simulink model "RBDmodel"  (R2023a)
settings: Solver=ode15s  StartTime=0.0  StopTime=4  FixedStep=0.0001  RelTol=1e-3  AbsTol=1e-3  EnableMultiTasking=on
model workspace (MAT data in the model file):
  C_Gimbal = 0.5
  C_IAP = 0.01
  IAP_Pa = 0
  K_Gimbal = 0
  K_IAP = 200
  LeftAbdominalMuscleForce = 0
  LeftBackMuscleForce = 0
  LeftTransverse1MuscleForce = 0
  LeftTransverse2MuscleForce = 0
  Moment_AR = 0
  Moment_FE = 7.5
  Moment_LB = 0
  RightAbdominalMuscleForce = 0
  RightBackMuscleForce = 0
  RightTransverse1MuscleForce = 0
  RightTransverse2MuscleForce = 0
  a = 1
  b = 1
  muscle_color = [0 0 1]
  muscle_radius = 1
undefined symbols (not defined in the file): X, Y, Z
libraries: nesl_utility x346, sm_lib x329, simulink_extras x33, checkpacklib x3, simulink x1
(part 1 of 12)
settings Model: PacingRate=0.110000  Creator=Siril TD  LastModifiedBy=siril
settings SolverCC: ZeroCrossAlgorithm=Adaptive  AutoInsertRateTranBlk=on
settings DataIOCC: LimitDataPoints=on  MaxDataPoints=50000  ReturnWorkspaceOutputsName=SDOSimTest_Log
settings OptimizationCC: LifeSpan=inf
settings DebuggingCC: IgnoredZcDiagnostic=none  UnconnectedInputMsg=warning  UnconnectedOutputMsg=warning  UnconnectedLineMsg=warning  AllowSymbolicDim=off  SFUnexpectedBacktrackingDiag=warning  SFNoUnconditionalDefaultTransitionDiag=warning  SFExecutionAtInitializationDiag=none  ArithmeticOperatorsInVariantConditions=warning
settings ModelReferenceCC: EnableRefExpFcnMdlSchedulingChecks=on
settings SFSimCC: SimUseLocalCustomCode=off  CustomCodeUndefinedFunction=UseInterfaceOnly
settings RTWCC: RTWUseLocalCustomCode=off  DLArmComputeVersion=19.05
settings CodeAppCC: StateflowObjectComments=on
settings GRTTargetCC: TargetLangStandard=C89/C90 (ANSI)
settings ConfigComp: CovMetricSettings=dw  CovSaveCumulativeToWorkspaceVar=on  CovSaveSingleToWorkspaceVar=on  CovExternalEMLEnable=off  CovSFcnEnable=off
settings SimscapeCC: SimscapeLogType=all  SimscapeLogSimulationStatistics=on  SimscapeLogDataHistory=10000

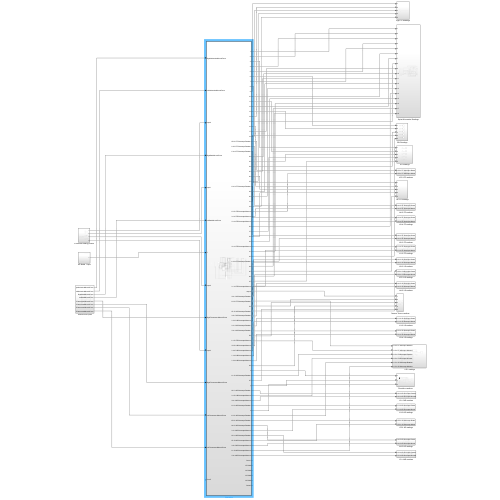
[thumbnail: Simulink's stored preview of the top-level diagram]
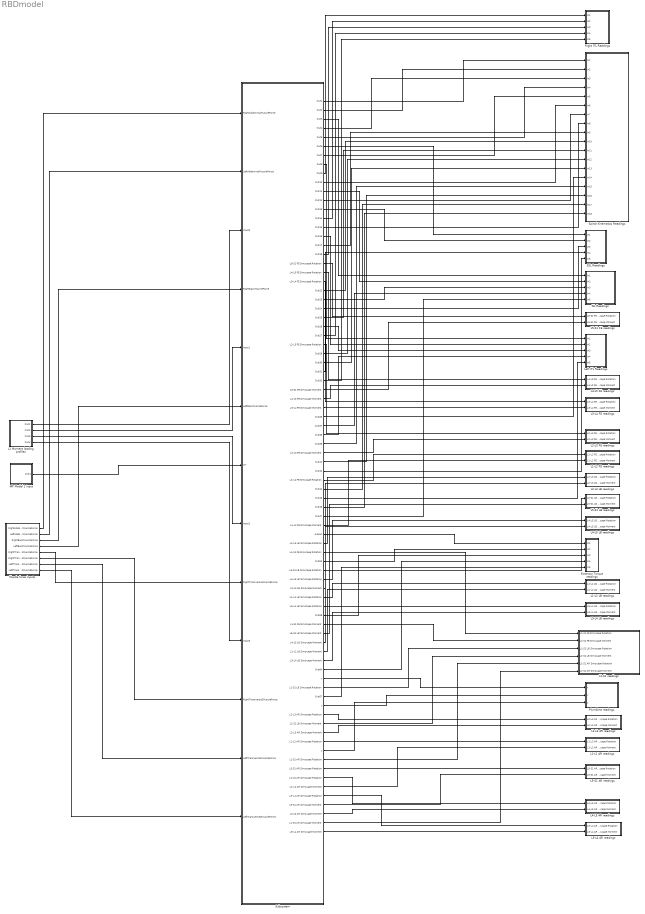
== system RBDmodel ==
  Extensor Torque readings : Subsystem
  IAP Model 1 input : Subsystem
  ISL Readings : Subsystem
  L1 Moment loading profiles : Subsystem
  L1-L2 AR readings : Subsystem
  L1-L2 FE readings : Subsystem
  L1-L2 LB readings : Subsystem
  L1-S1 readings : Subsystem
  L2-L3 AR readings : Subsystem
  L2-L3 FE readings : Subsystem
  L2-L3 LB readings : Subsystem
  L3-L4 AR readings : Subsystem
  L3-L4 FE readings : Subsystem
  L3-L4 LB readings : Subsystem
  L4-L5 AR readings : Subsystem
  L4-L5 FE readings : Subsystem
  L4-L5 LB readings : Subsystem
  L5-S1 AR readings : Subsystem
  L5-S1 FE readings : Subsystem
  L5-S1 LB readings : Subsystem
  Left ITL Readings : Subsystem
  Muscle force inputs : Subsystem
  Plumbline readings : Subsystem
  Right ITL Readings : Subsystem
  SSL Readings : Subsystem
  Spinal Kinematics Readings : Subsystem
  Subsystem : Subsystem  TreatAsAtomicUnit=on
  wires:
  Subsystem/20(L4-L5 FE Simscape Rotation) -> L4-L5 FE readings/1(L4-L5 FE Simscape Rotation)
  Subsystem/67(Out67) -> Extensor Torque readings/5(In5)
  Muscle force inputs/4(LeftBackMuscleForce) -> Subsystem/6(LeftBackMuscleForce)
  Muscle force inputs/3(RightBackMuscleForce) -> Subsystem/4(RightBackMuscleForce)
  L1 Moment loading profiles/1(Out1) -> Subsystem/3(input0)
  Subsystem/31(Out31) -> SSL Readings/4(In4)
  Subsystem/81(L1-S1 AR Simscape Moment) -> L1-S1 readings/6(L1-S1 AR Simscape Moment)
  Subsystem/56(L1-L2 LB Simscape Rotation) -> L1-L2 LB readings/1(L1-L2 LB Simscape Rotation)
  L1 Moment loading profiles/2(Out2) -> Subsystem/5(input1)
  L1 Moment loading profiles/3(Out3) -> Subsystem/8(input2)
  Subsystem/50(L2-L3 LB Simscape Rotation) -> L2-L3 LB readings/1(L2-L3 LB Simscape Rotation)
  Subsystem/6(Out6) -> SSL Readings/1(In1)
  L1 Moment loading profiles/4(Out4) -> Subsystem/10(input3)
  Muscle force inputs/1(RightAbdominalMuscleForce) -> Subsystem/1(RightAbdominalMuscleForce)
  Subsystem/16(Out16) -> Left ITL Readings/2(In2)
  IAP Model 1 input/1(Out1) -> Subsystem/7(In7)
  Muscle force inputs/2(LeftAbdominalMuscleForce) -> Subsystem/2(LeftAbdominalMuscleForce)
  Muscle force inputs/5(RightTransverse1MuscleForce) -> Subsystem/9(RightTransverse1MuscleForce)
  Muscle force inputs/6(RightTransverse2MuscleForce) -> Subsystem/11(RightTransverse2MuscleForce)
  Subsystem/62(L1-L2 LB Simscape Moment) -> L1-L2 LB readings/2(L1-L2 LB Simscape Moment)
  Muscle force inputs/8(LeftTransverse2MuscleForce) -> Subsystem/13(LeftTransverse2MuscleForce)
  Muscle force inputs/7(LeftTransverse1MuscleForce) -> Subsystem/12(LeftTransverse1MuscleForce)
  Subsystem/63(L3-L4 LB Simscape Moment) -> L3-L4 LB readings/2(L3-L4 LB Simscape Moment)
  Subsystem/1(Out1) -> Spinal Kinematics Readings/1(In1)
  Subsystem/30(Out30) -> Spinal Kinematics Readings/13(In13)
  Subsystem/2(Out2) -> Spinal Kinematics Readings/2(In2)
  Subsystem/13(Out13) -> SSL Readings/2(In2)
  Subsystem/21(L3-L4 FE Simscape Rotation) -> L3-L4 FE readings/1(L3-L4 FE Simscape Rotation)
  Subsystem/3(Out3) -> ISL Readings/1(In1)
  Subsystem/44(Out44) -> Spinal Kinematics Readings/17(In17)
  Subsystem/25(Out25) -> Spinal Kinematics Readings/11(In11)
  Subsystem/79(L5-S1 AR Simscape Moment) -> L5-S1 AR readings/2(L5-S1 AR Simscape Moment)
  Subsystem/4(Out4) -> Spinal Kinematics Readings/3(In3)
  Subsystem/5(Out5) -> Spinal Kinematics Readings/4(In4)
  Subsystem/77(L1-L2 AR Simscape Moment) -> L1-L2 AR readings/2(L1-L2 AR Simscape Moment)
  Subsystem/36(Out36) -> Spinal Kinematics Readings/14(In14)
  Subsystem/78(L3-L4 AR Simscape Rotation) -> L3-L4 AR readings/1(L3-L4 AR Simscape Rotation)
  Subsystem/26(Out26) -> Left ITL Readings/3(In3)
  Subsystem/7(Out7) -> Spinal Kinematics Readings/5(In5)
  Subsystem/18(Out18) -> Right ITL Readings/3(In3)
  Subsystem/8(Out8) -> Left ITL Readings/1(In1)
  Subsystem/9(Out9) -> Right ITL Readings/1(In1)
  Subsystem/10(Out10) -> Spinal Kinematics Readings/6(In6)
  Subsystem/11(Out11) -> ISL Readings/2(In2)
  Subsystem/12(Out12) -> Spinal Kinematics Readings/7(In7)
  Subsystem/38(Out38) -> Left ITL Readings/4(In4)
  Subsystem/14(Out14) -> Right ITL Readings/2(In2)
  Subsystem/15(Out15) -> Spinal Kinematics Readings/8(In8)
  Subsystem/17(Out17) -> Spinal Kinematics Readings/9(In9)
  Subsystem/27(Out27) -> Right ITL Readings/4(In4)
  Subsystem/19(L5-S1 FE Simscape Rotation) -> L5-S1 FE readings/1(L5-S1 FE Simscape Rotation)
  Subsystem/22(Out22) -> Spinal Kinematics Readings/10(In10)
  Subsystem/33(L5-S1 FE Simscape Moment) -> L5-S1 FE readings/2(L5-S1 FE Simscape Moment)
  Subsystem/23(Out23) -> ISL Readings/3(In3)
  Subsystem/45(Out45) -> Left ITL Readings/5(In5)
  Subsystem/24(Out24) -> SSL Readings/3(In3)
  Subsystem/28(L2-L3 FE Simscape Rotation) -> L2-L3 FE readings/1(L2-L3 FE Simscape Rotation)
  Subsystem/29(Out29) -> Spinal Kinematics Readings/12(In12)
  Subsystem/32(Out32) -> Right ITL Readings/5(In5)
  Subsystem/34(L4-L5 FE Simscape Moment) -> L4-L5 FE readings/2(L4-L5 FE Simscape Moment)
  Subsystem/59(L1-S1 FE Simscape Moment) -> L1-S1 readings/2(L1-S1 FE Simscape Moment)
  Subsystem/35(L3-L4 FE Simscape Moment) -> L3-L4 FE readings/2(L3-L4 FE Simscape Moment)
  Subsystem/37(Out37) -> ISL Readings/4(In4)
  Subsystem/51(L1-S1 FE Simscape Rotation) -> L1-S1 readings/1(L1-S1 FE Simscape Rotation)
  Subsystem/39(Out39) -> Spinal Kinematics Readings/15(In15)
  Subsystem/40(L2-L3 FE Simscape Moment) -> L2-L3 FE readings/2(L2-L3 FE Simscape Moment)
  Subsystem/41(Out41) -> Spinal Kinematics Readings/16(In16)
  Subsystem/42(Out42) -> SSL Readings/5(In5)
  Subsystem/43(L1-L2 FE Simscape Rotation) -> L1-L2 FE readings/1(L1-L2 FE Simscape Rotation)
  Subsystem/46(Out46) -> Spinal Kinematics Readings/18(In18)
  Subsystem/47(Out47) -> ISL Readings/5(In5)
  Subsystem/48(L1-L2 FE Simscape Moment) -> L1-L2 FE readings/2(L1-L2 FE Simscape Moment)
  Subsystem/49(output) -> Extensor Torque readings/1(In1)
  Subsystem/52(Out52) -> Extensor Torque readings/2(In2)
  Subsystem/68(y) -> Plumbline readings/2(y)
  Subsystem/53(L5-S1 LB Simscape Rotation) -> L5-S1 LB readings/1(L5-S1 LB Simscape Rotation)
  Subsystem/54(L4-L5 LB Simscape Rotation) -> L4-L5 LB readings/1(L4-L5 LB Simscape Rotation)
  Subsystem/55(L2-L3 LB Simscape Moment) -> L2-L3 LB readings/2(L2-L3 LB Simscape Moment)
  Subsystem/57(L3-L4 LB Simscape Rotation) -> L3-L4 LB readings/1(L3-L4 LB Simscape Rotation)
  Subsystem/58(Out58) -> Extensor Torque readings/3(In3)
  Subsystem/60(L5-S1 LB Simscape Moment) -> L5-S1 LB readings/2(L5-S1 LB Simscape Moment)
  Subsystem/61(L4-L5 LB Simscape Moment) -> L4-L5 LB readings/2(L4-L5 LB Simscape Moment)
  Subsystem/64(Out64) -> Extensor Torque readings/4(In4)
  Subsystem/65(x) -> Plumbline readings/1(x)
  Subsystem/66(L1-S1 LB Simscape Rotation) -> L1-S1 readings/3(L1-S1 LB Simscape Rotation)
  Subsystem/69(L2-L3 AR Simscape Rotation) -> L2-L3 AR readings/1(L2-L3 AR Simscape Rotation)
  Subsystem/70(L1-S1 LB Simscape Moment) -> L1-S1 readings/4(L1-S1 LB Simscape Moment)
  Subsystem/71(L2-L3 AR Simscape Moment) -> L2-L3 AR readings/2(L2-L3 AR Simscape Moment)
  Subsystem/72(L1-L2 AR Simscape Rotation) -> L1-L2 AR readings/1(L1-L2 AR Simscape Rotation)
  Subsystem/73(z) -> Plumbline readings/3(z)
  Subsystem/74(L1-S1 AR Simscape Rotation) -> L1-S1 readings/5(L1-S1 AR Simscape Rotation)
  Subsystem/75(L5-S1 AR Simscape Rotation) -> L5-S1 AR readings/1(L5-S1 AR Simscape Rotation)
  Subsystem/76(L4-L5 AR Simscape Rotation) -> L4-L5 AR readings/1(L4-L5 AR Simscape Rotation)
  Subsystem/80(L4-L5 AR Simscape Moment) -> L4-L5 AR readings/2(L4-L5 AR Simscape Moment)
  Subsystem/82(L3-L4 AR Simscape Moment) -> L3-L4 AR readings/2(L3-L4 AR Simscape Moment)

== system RBDmodel/Extensor Torque readings ==
  In1 : Inport
  In2 : Inport  Port=2
  In3 : Inport  Port=3
  In4 : Inport  Port=4
  In5 : Inport  Port=5
  Display{,1..4} (5 alike) : Display
      settings: Decimation=2
  Gain{9,11..14} (5 alike) : Gain
  IAP Extensor Torque at L1-L2 : Scope
  IAP Extensor Torque at L2-L3 (reported) : Scope
  IAP Extensor Torque at L3-L4 : Scope
  IAP Extensor Torque at L4-L5 : Scope
  IAP Extensor Torque at L5-S1 : Scope
  wires:
  Gain11/1 -> Display1/1
  Gain9/1 -> Display/1
  In5/1 -> Gain14/1, IAP Extensor Torque at L5-S1/1
  In2/1 -> Gain9/1, IAP Extensor Torque at L2-L3 (reported)/1
  Gain12/1 -> Display2/1
  In4/1 -> Gain13/1, IAP Extensor Torque at L4-L5/1
  In3/1 -> Gain12/1, IAP Extensor Torque at L3-L4/1
  Gain13/1 -> Display3/1
  In1/1 -> Gain11/1, IAP Extensor Torque at L1-L2/1
  Gain14/1 -> Display4/1

== system RBDmodel/IAP Model 1 input ==
  Constant96 : Constant  Value=IAP_Pa
  Out1 : Outport
  wires:
  Constant96/1 -> Out1/1

== system RBDmodel/ISL Readings ==
  In1 : Inport
  In2 : Inport  Port=2
  In3 : Inport  Port=3
  In4 : Inport  Port=4
  In5 : Inport  Port=5
  L1-L2 ISL force : Scope
  L2-L3 ISL force : Scope
  L3-L4 ISL force : Scope
  L4-L5 ISL force : Scope
  L5-S1 ISL force : Scope
  wires:
  In4/1 -> L5-S1 ISL force/1
  In2/1 -> L2-L3 ISL force/1
  In1/1 -> L1-L2 ISL force/1
  In3/1 -> L3-L4 ISL force/1
  In5/1 -> L4-L5 ISL force/1

== system RBDmodel/L1 Moment loading profiles ==
  Gain10 : Gain  Gain=-1
  Horizontal force at T1 : simulink/Sources/Ramp  slope=0  start=0  InitialOutput=0
  Moment_AR : Sin  Amplitude=Moment_AR  SampleTime=0
  Moment_FE : Sin  Amplitude=-Moment_FE  SampleTime=0
  Moment_LB : Sin  Amplitude=-Moment_LB  SampleTime=0
  Scope2 : Scope
  Out1 : Outport
  Out2 : Outport  Port=2
  Out3 : Outport  Port=3
  Out4 : Outport  Port=4
  wires:
  Gain10/1 -> Scope2/1
  Horizontal force at T1/1 -> Out4/1
  Moment_LB/1 -> Out2/1
  Moment_AR/1 -> Out1/1
  Moment_FE/1 -> Gain10/1, Out3/1

== system RBDmodel/L1-L2 AR readings ==
  L1-L2 AR Simscape Rotation : Inport
  L1-L2 AR Simscape Moment : Inport  Port=2
  L1-L2 AR Moment : Scope
  L1-L2 AR Rotation : Scope
  L1-L2 AR Simscape : Record  FileSettingsInternal="{\"entries\":[{\"content\":{\"excelSettings\":{\"content\":{},\"type\":\"Streamout.ExcelSettings\"}},\"type\":\"Streamout.FileSettingStorage\",\"uuid\":\"b28dc066-991e-4613-a00d-d29ff6d798a1\"}],\"packageUris\":[\"http://schema.mathworks.com/mf0/streamout_blocks/R2020a\"],\"version\":\"1.0\"}"  Layout=[1 1]  SignalsInternal="{\"entries\":[{\"content\":{\"signals\":[{\"content\":{\"blockPath\":[\"RBDmodel/L1-L2 AR readings/L1-L2 AR Simscape\"],\"dimensions\":[1],\"domain\":\"RBDmodel/L1-L2 AR readings/L1-L2 AR Simscape\",\"lineColor\":\"#ff6929\",\"port\":1,\"sid\":[\"\"],\"signalID\":1360,\"signalName\":\"L1-L2 AR Simscape Rotation\"},\"type\":\"RecordBlkView.Signal\",\"uuid\":\"8ba76c58-794a-4c9e-a7b1-df05cf77fcb8\"},{\"content\":{\"blockPath\":[\"RBDmodel/L1-L2 AR readings/L1-L2 AR Simscape\"],\"dimensions\":[1],\"domain\":\"RBDmodel/L1-L2 AR readings/L1-L2 AR Simscape\",\"lineColor\":\"#b746ff\",\"port\":2,\"sid\":[\"\"],\"signalID\":1364,\"signalName\":\"L1-L2 AR Simscape Moment\"},\"type\":\"RecordBlkView.Signal\",\"uuid\":\"7d4a0f01-01c2-4817-9b83-8632446fab25\"}]},\"type\":\"RecordBlkView.InputSignals\",\"uuid\":\"3a315800-566e-4bdd-9ec3-69dc347d5a26\"}],\"packageUris\":[\"http://schema.mathworks.com/mf0/streamout_blocks/R2020a\"],\"version\":\"1.0\"}"  VisualizationBindings="{\"xyplotplugin\":{\"info\":[{\"series\":[],\"subplotID\":1}]}}"  CompatibilityTag=XY
  wires:
  L1-L2 AR Simscape Rotation/1 -> L1-L2 AR Simscape/1, L1-L2 AR Rotation/1
  L1-L2 AR Simscape Moment/1 -> L1-L2 AR Simscape/2, L1-L2 AR Moment/1

== system RBDmodel/L1-L2 FE readings ==
  L1-L2 FE Simscape Rotation : Inport
  L1-L2 FE Simscape Moment : Inport  Port=2
  L1-L2 FE Moment : Scope
  L1-L2 FE Rotation : Scope
  L1-L2 FE Simscape : Record  FileSettingsInternal="{\"entries\":[{\"content\":{\"excelSettings\":{\"content\":{},\"type\":\"Streamout.ExcelSettings\"}},\"type\":\"Streamout.FileSettingStorage\",\"uuid\":\"8ce7ea1e-727d-4085-a2f9-c3a4a6f5bb0a\"}],\"packageUris\":[\"http://schema.mathworks.com/mf0/streamout_blocks/R2020a\"],\"version\":\"1.0\"}"  Layout=[1 1]  SignalsInternal="{\"entries\":[{\"content\":{\"signals\":[{\"content\":{\"blockPath\":[\"RBDmodel/L1-L2 FE readings/L1-L2 FE Simscape\"],\"dimensions\":[1],\"domain\":\"RBDmodel/L1-L2 FE readings/L1-L2 FE Simscape\",\"lineColor\":\"#64d413\",\"port\":1,\"sid\":[\"\"],\"signalID\":1368,\"signalName\":\"L1-L2 FE Simscape Rotation\"},\"type\":\"RecordBlkView.Signal\",\"uuid\":\"2003be24-72ea-4258-88d8-cae005e22d9e\"},{\"content\":{\"blockPath\":[\"RBDmodel/L1-L2 FE readings/L1-L2 FE Simscape\"],\"dimensions\":[1],\"domain\":\"RBDmodel/L1-L2 FE readings/L1-L2 FE Simscape\",\"lineColor\":\"#ff13a6\",\"port\":2,\"sid\":[\"\"],\"signalID\":1372,\"signalName\":\"L1-L2 FE Simscape Moment\"},\"type\":\"RecordBlkView.Signal\",\"uuid\":\"2512a7a8-a368-412a-aefb-8db868f0d60c\"}]},\"type\":\"RecordBlkView.InputSignals\",\"uuid\":\"ac10ff46-4b91-49cb-b675-363e0bf05791\"}],\"packageUris\":[\"http://schema.mathworks.com/mf0/streamout_blocks/R2020a\"],\"version\":\"1.0\"}"  VisualizationBindings="{\"xyplotplugin\":{\"info\":[{\"series\":[],\"subplotID\":1}]}}"  CompatibilityTag=XY
  wires:
  L1-L2 FE Simscape Rotation/1 -> L1-L2 FE Simscape/1, L1-L2 FE Rotation/1
  L1-L2 FE Simscape Moment/1 -> L1-L2 FE Simscape/2, L1-L2 FE Moment/1

== system RBDmodel/L1-L2 LB readings ==
  L1-L2 LB Simscape Rotation : Inport
  L1-L2 LB Simscape Moment : Inport  Port=2
  L1-L2 LB Moment : Scope
  L1-L2 LB Rotation : Scope
  L1-L2 LB Simscape : Record  FileSettingsInternal="{\"entries\":[{\"content\":{\"excelSettings\":{\"content\":{},\"type\":\"Streamout.ExcelSettings\"}},\"type\":\"Streamout.FileSettingStorage\",\"uuid\":\"f91b6da8-1a5e-44a2-9c0b-2edd10b764e6\"}],\"packageUris\":[\"http://schema.mathworks.com/mf0/streamout_blocks/R2020a\"],\"version\":\"1.0\"}"  Layout=[1 1]  SignalsInternal="{\"entries\":[{\"content\":{\"signals\":[{\"content\":{\"blockPath\":[\"RBDmodel/L1-L2 LB readings/L1-L2 LB Simscape\"],\"dimensions\":[1],\"domain\":\"RBDmodel/L1-L2 LB readings/L1-L2 LB Simscape\",\"lineColor\":\"#fe330a\",\"port\":1,\"sid\":[\"\"],\"signalID\":1376,\"signalName\":\"L1-L2 LB Simscape Rotation\"},\"type\":\"RecordBlkView.Signal\",\"uuid\":\"685ac858-44fe-41ed-9867-a98cbe032e53\"},{\"content\":{\"blockPath\":[\"RBDmodel/L1-L2 LB readings/L1-L2 LB Simscape\"],\"dimensions\":[1],\"domain\":\"RBDmodel/L1-L2 LB readings/L1-L2 LB Simscape\",\"lineColor\":\"#22b573\",\"port\":2,\"sid\":[\"\"],\"signalID\":1380,\"signalName\":\"L1-L2 LB Simscape Moment\"},\"type\":\"RecordBlkView.Signal\",\"uuid\":\"d180cd7c-5a37-42c6-8969-9ba706f80bc0\"}]},\"type\":\"RecordBlkView.InputSignals\",\"uuid\":\"702aeb74-2cc2-4c6d-93f9-3cbe42c69f5a\"}],\"packageUris\":[\"http://schema.mathworks.com/mf0/streamout_blocks/R2020a\"],\"version\":\"1.0\"}"  VisualizationBindings="{\"xyplotplugin\":{\"info\":[{\"series\":[],\"subplotID\":1}]}}"  CompatibilityTag=XY
  wires:
  L1-L2 LB Simscape Moment/1 -> L1-L2 LB Simscape/2, L1-L2 LB Moment/1
  L1-L2 LB Simscape Rotation/1 -> L1-L2 LB Simscape/1, L1-L2 LB Rotation/1

== system RBDmodel/L1-S1 readings ==
  L1-S1 FE Simscape Rotation : Inport
  L1-S1 FE Simscape Moment : Inport  Port=2
  L1-S1 LB Simscape Rotation : Inport  Port=3
  L1-S1 LB Simscape Moment : Inport  Port=4
  L1-S1 AR Simscape Rotation : Inport  Port=5
  L1-S1 AR Simscape Moment : Inport  Port=6
  Check Flexion Angle : checkpacklib/Check Custom Bounds  InstantiateOnLoad=on  enabled=off  stopWhenAssertionFail=off  export=off  ViewDlgPos=[100 200 510 390]  OpenViewOnLoad=off  LaunchViewOnOpen=off  TimeUnits=seconds  EnableUpperBound=on  UpperBoundTimes=[5 10]  UpperBoundAmplitudes=[51 51];  EnableLowerBound=on  LowerBoundTimes=[6 10]  LowerBoundAmplitudes=[49 49];
      settings: LibrarySourceBlock=sdolib/Signal Constraints/Check Custom Bounds
  L1-S1 AR Rotation : Scope
  L1-S1 AR Simscape : Record  FileSettingsInternal="{\"entries\":[{\"content\":{\"excelSettings\":{\"content\":{},\"type\":\"Streamout.ExcelSettings\"}},\"type\":\"Streamout.FileSettingStorage\",\"uuid\":\"b954e3b6-b992-4288-8e9e-83c0e0eed84f\"}],\"packageUris\":[\"http://schema.mathworks.com/mf0/streamout_blocks/R2020a\"],\"version\":\"1.0\"}"  Layout=[1 1]  SignalsInternal="{\"entries\":[{\"content\":{\"signals\":[{\"content\":{\"blockPath\":[\"RBDmodel/L1-S1 readings/L1-S1 AR Simscape\"],\"dimensions\":[1,1],\"domain\":\"RBDmodel/L1-S1 readings/L1-S1 AR Simscape\",\"lineColor\":\"#edb120\",\"port\":1,\"sid\":[\"\"],\"signalID\":1392,\"signalName\":\"L1-S1 AR Simscape Rotation\"},\"type\":\"RecordBlkView.Signal\",\"uuid\":\"2e278b6b-2be8-4276-afd2-a0bb5f9fc5b0\"},{\"content\":{\"blockPath\":[\"RBDmodel/L1-S1 readings/L1-S1 AR Simscape\"],\"dimensions\":[1],\"domain\":\"RBDmodel/L1-S1 readings/L1-S1 AR Simscape\",\"lineColor\":\"#7e2f8e\",\"port\":2,\"sid\":[\"\"],\"signalID\":1396,\"signalName\":\"L1-S1 AR Simscape Moment\"},\"type\":\"RecordBlkView.Signal\",\"uuid\":\"2c4962eb-e85a-4893-ad71-a0813a35683c\"}]},\"type\":\"RecordBlkView.InputSignals\",\"uuid\":\"a7594377-7e8f-4472-89c7-d235376936c0\"}],\"packageUris\":[\"http://schema.mathworks.com/mf0/streamout_blocks/R2020a\"],\"version\":\"1.0\"}"  VisualizationBindings="{\"xyplotplugin\":{\"info\":[{\"series\":[],\"subplotID\":1}]}}"  CompatibilityTag=XY
  L1-S1 AR when LB loading : Record  FileSettingsInternal="{\"entries\":[{\"content\":{\"excelSettings\":{\"content\":{},\"type\":\"Streamout.ExcelSettings\"}},\"type\":\"Streamout.FileSettingStorage\",\"uuid\":\"7c9a55b9-26e2-4dee-8ab6-75e3d662341a\"}],\"packageUris\":[\"http://schema.mathworks.com/mf0/streamout_blocks/R2020a\"],\"version\":\"1.0\"}"  Layout=[1 1]  SignalsInternal="{\"entries\":[{\"content\":{\"signals\":[{\"content\":{\"blockPath\":[\"RBDmodel/L1-S1 readings/L1-S1 AR when LB loading\"],\"dimensions\":[1,1],\"domain\":\"RBDmodel/L1-S1 readings/L1-S1 AR when LB loading\",\"lineColor\":\"#77ac30\",\"port\":1,\"sid\":[\"\"],\"signalID\":1400,\"signalName\":\"L1-S1 AR Simscape Rotation\"},\"type\":\"RecordBlkView.Signal\",\"uuid\":\"236197de-69c7-448b-8f27-f03d1694973f\"},{\"content\":{\"blockPath\":[\"RBDmodel/L1-S1 readings/L1-S1 AR when LB loading\"],\"dimensions\":[1],\"domain\":\"RBDmodel/L1-S1 readings/L1-S1 AR when LB loading\",\"lineColor\":\"#4dbeee\",\"port\":2,\"sid\":[\"\"],\"signalID\":1404,\"signalName\":\"L1-S1 LB Simscape Moment\"},\"type\":\"RecordBlkView.Signal\",\"uuid\":\"affd1b11-9ea1-4649-962a-1b25dd418c96\"}]},\"type\":\"RecordBlkView.InputSignals\",\"uuid\":\"d23c6d54-c8cf-463c-b3c1-026604afceae\"}],\"packageUris\":[\"http://schema.mathworks.com/mf0/streamout_blocks/R2020a\"],\"version\":\"1.0\"}"  VisualizationBindings="{\"xyplotplugin\":{\"info\":[{\"series\":[],\"subplotID\":1}]}}"  CompatibilityTag=XY
  L1-S1 FE Rotation : Scope
  L1-S1 FE Simscape : Record  FileSettingsInternal="{\"entries\":[{\"content\":{\"excelSettings\":{\"content\":{},\"type\":\"Streamout.ExcelSettings\"}},\"type\":\"Streamout.FileSettingStorage\",\"uuid\":\"4277ec63-d6bc-434d-a603-e60f5b770cfc\"}],\"packageUris\":[\"http://schema.mathworks.com/mf0/streamout_blocks/R2020a\"],\"version\":\"1.0\"}"  Layout=[1 1]  SignalsInternal="{\"entries\":[{\"content\":{\"signals\":[{\"content\":{\"blockPath\":[\"RBDmodel/L1-S1 readings/L1-S1 FE Simscape\"],\"dimensions\":[1,1],\"domain\":\"RBDmodel/L1-S1 readings/L1-S1 FE Simscape\",\"lineColor\":\"#0072bd\",\"port\":1,\"sid\":[\"\"],\"signalID\":1384,\"signalName\":\"L1-S1 FE Simscape Rotation\"},\"type\":\"RecordBlkView.Signal\",\"uuid\":\"95e268ca-b23d-4342-a972-90dd635bc70e\"},{\"content\":{\"blockPath\":[\"RBDmodel/L1-S1 readings/L1-S1 FE Simscape\"],\"dimensions\":[1],\"domain\":\"RBDmodel/L1-S1 readings/L1-S1 FE Simscape\",\"lineColor\":\"#d95319\",\"port\":2,\"sid\":[\"\"],\"signalID\":1388,\"signalName\":\"L1-S1 FE Simscape Moment\"},\"type\":\"RecordBlkView.Signal\",\"uuid\":\"382e9f89-fefe-4a91-94ad-6604e6821858\"}]},\"type\":\"RecordBlkView.InputSignals\",\"uuid\":\"562346bb-41eb-431e-8171-f017e49566b0\"}],\"packageUris\":[\"http://schema.mathworks.com/mf0/streamout_blocks/R2020a\"],\"version\":\"1.0\"}"  VisualizationBindings="{\"xyplotplugin\":{\"info\":[{\"series\":[],\"subplotID\":1}]}}"  CompatibilityTag=XY
  L1-S1 LB Rotation : Scope
  L1-S1 LB Simscape : Record  FileSettingsInternal="{\"entries\":[{\"content\":{\"excelSettings\":{\"content\":{},\"type\":\"Streamout.ExcelSettings\"}},\"type\":\"Streamout.FileSettingStorage\",\"uuid\":\"d051a5cc-fb2e-466c-bd05-561f4ba50a96\"}],\"packageUris\":[\"http://schema.mathworks.com/mf0/streamout_blocks/R2020a\"],\"version\":\"1.0\"}"  Layout=[1 1]  SignalsInternal="{\"entries\":[{\"content\":{\"signals\":[{\"content\":{\"blockPath\":[\"RBDmodel/L1-S1 readings/L1-S1 LB Simscape\"],\"dimensions\":[1,1],\"domain\":\"RBDmodel/L1-S1 readings/L1-S1 LB Simscape\",\"lineColor\":\"#a2142f\",\"port\":1,\"sid\":[\"\"],\"signalID\":1408,\"signalName\":\"L1-S1 LB Simscape Rotation\"},\"type\":\"RecordBlkView.Signal\",\"uuid\":\"18954a4d-601c-4dd8-9b7b-399a90aadc1e\"},{\"content\":{\"blockPath\":[\"RBDmodel/L1-S1 readings/L1-S1 LB Simscape\"],\"dimensions\":[1],\"domain\":\"RBDmodel/L1-S1 readings/L1-S1 LB Simscape\",\"lineColor\":\"#139fff\",\"port\":2,\"sid\":[\"\"],\"signalID\":1412,\"signalName\":\"L1-S1 LB Simscape Moment\"},\"type\":\"RecordBlkView.Signal\",\"uuid\":\"a6ca627e-51ce-4d8f-9c49-1dfe1e8cd011\"}]},\"type\":\"RecordBlkView.InputSignals\",\"uuid\":\"052f090c-a55b-4592-abd6-786af4de0160\"}],\"packageUris\":[\"http://schema.mathworks.com/mf0/streamout_blocks/R2020a\"],\"version\":\"1.0\"}"  VisualizationBindings="{\"xyplotplugin\":{\"info\":[{\"series\":[],\"subplotID\":1}]}}"  CompatibilityTag=XY
  wires:
  L1-S1 LB Simscape Rotation/1 -> L1-S1 LB Simscape/1, L1-S1 LB Rotation/1
  L1-S1 FE Simscape Rotation/1 -> Check Flexion Angle/1, L1-S1 FE Rotation/1, L1-S1 FE Simscape/1
  L1-S1 AR Simscape Rotation/1 -> L1-S1 AR when LB loading/1, L1-S1 AR Rotation/1, L1-S1 AR Simscape/1
  L1-S1 LB Simscape Moment/1 -> L1-S1 LB Simscape/2, L1-S1 AR when LB loading/2
  L1-S1 FE Simscape Moment/1 -> L1-S1 FE Simscape/2
  L1-S1 AR Simscape Moment/1 -> L1-S1 AR Simscape/2

== system RBDmodel/L2-L3 AR readings ==
  L2-L3 AR Simscape Rotation : Inport
  L2-L3 AR Simscape Moment : Inport  Port=2
  L2-L3 AR Moment : Scope
  L2-L3 AR Rotation : Scope
  L2-L3 AR Simscape : Record  FileSettingsInternal="{\"entries\":[{\"content\":{\"excelSettings\":{\"content\":{},\"type\":\"Streamout.ExcelSettings\"}},\"type\":\"Streamout.FileSettingStorage\",\"uuid\":\"1b3dca45-e25d-4c43-83f1-4bff6aa87f96\"}],\"packageUris\":[\"http://schema.mathworks.com/mf0/streamout_blocks/R2020a\"],\"version\":\"1.0\"}"  Layout=[1 1]  SignalsInternal="{\"entries\":[{\"content\":{\"signals\":[{\"content\":{\"blockPath\":[\"RBDmodel/L2-L3 AR readings/L2-L3 AR Simscape\"],\"dimensions\":[1],\"domain\":\"RBDmodel/L2-L3 AR readings/L2-L3 AR Simscape\",\"lineColor\":\"#ff6929\",\"port\":1,\"sid\":[\"\"],\"signalID\":1416,\"signalName\":\"L2-L3 AR Simscape Rotation\"},\"type\":\"RecordBlkView.Signal\",\"uuid\":\"834c48d4-b959-4b71-a361-c754261b6a00\"},{\"content\":{\"blockPath\":[\"RBDmodel/L2-L3 AR readings/L2-L3 AR Simscape\"],\"dimensions\":[1],\"domain\":\"RBDmodel/L2-L3 AR readings/L2-L3 AR Simscape\",\"lineColor\":\"#b746ff\",\"port\":2,\"sid\":[\"\"],\"signalID\":1420,\"signalName\":\"L2-L3 AR Simscape Moment\"},\"type\":\"RecordBlkView.Signal\",\"uuid\":\"24cf7c8b-c1f2-4173-9894-3cad208cfe16\"}]},\"type\":\"RecordBlkView.InputSignals\",\"uuid\":\"c1cde1dc-d4fe-4b90-870d-696a5867ce42\"}],\"packageUris\":[\"http://schema.mathworks.com/mf0/streamout_blocks/R2020a\"],\"version\":\"1.0\"}"  VisualizationBindings="{\"xyplotplugin\":{\"info\":[{\"series\":[],\"subplotID\":1}]}}"  CompatibilityTag=XY
  wires:
  L2-L3 AR Simscape Rotation/1 -> L2-L3 AR Simscape/1, L2-L3 AR Rotation/1
  L2-L3 AR Simscape Moment/1 -> L2-L3 AR Simscape/2, L2-L3 AR Moment/1

== system RBDmodel/L2-L3 FE readings ==
  L2-L3 FE Simscape Rotation : Inport
  L2-L3 FE Simscape Moment : Inport  Port=2
  L2-L3 FE Moment : Scope
  L2-L3 FE Rotation : Scope
  L2-L3 FE Simscape : Record  FileSettingsInternal="{\"entries\":[{\"content\":{\"excelSettings\":{\"content\":{},\"type\":\"Streamout.ExcelSettings\"}},\"type\":\"Streamout.FileSettingStorage\",\"uuid\":\"a8dbeb5b-ff1f-49c5-807a-ed83070a13e0\"}],\"packageUris\":[\"http://schema.mathworks.com/mf0/streamout_blocks/R2020a\"],\"version\":\"1.0\"}"  Layout=[1 1]  SignalsInternal="{\"entries\":[{\"content\":{\"signals\":[{\"content\":{\"blockPath\":[\"RBDmodel/L2-L3 FE readings/L2-L3 FE Simscape\"],\"dimensions\":[1],\"domain\":\"RBDmodel/L2-L3 FE readings/L2-L3 FE Simscape\",\"lineColor\":\"#64d413\",\"port\":1,\"sid\":[\"\"],\"signalID\":1424,\"signalName\":\"L2-L3 FE Simscape Rotation\"},\"type\":\"RecordBlkView.Signal\",\"uuid\":\"e9322bc5-4954-459f-83fa-eebb47a259c0\"},{\"content\":{\"blockPath\":[\"RBDmodel/L2-L3 FE readings/L2-L3 FE Simscape\"],\"dimensions\":[1],\"domain\":\"RBDmodel/L2-L3 FE readings/L2-L3 FE Simscape\",\"lineColor\":\"#ff13a6\",\"port\":2,\"sid\":[\"\"],\"signalID\":1428,\"signalName\":\"L2-L3 FE Simscape Moment\"},\"type\":\"RecordBlkView.Signal\",\"uuid\":\"26ccf091-bec1-45f3-9b99-f9ea3151294d\"}]},\"type\":\"RecordBlkView.InputSignals\",\"uuid\":\"80a7115b-5c25-41a3-8ec9-9dbb82154804\"}],\"packageUris\":[\"http://schema.mathworks.com/mf0/streamout_blocks/R2020a\"],\"version\":\"1.0\"}"  VisualizationBindings="{\"xyplotplugin\":{\"info\":[{\"series\":[],\"subplotID\":1}]}}"  CompatibilityTag=XY
  wires:
  L2-L3 FE Simscape Rotation/1 -> L2-L3 FE Simscape/1, L2-L3 FE Rotation/1
  L2-L3 FE Simscape Moment/1 -> L2-L3 FE Simscape/2, L2-L3 FE Moment/1

== system RBDmodel/L2-L3 LB readings ==
  L2-L3 LB Simscape Rotation : Inport
  L2-L3 LB Simscape Moment : Inport  Port=2
  L2-L3 LB Moment : Scope
  L2-L3 LB Rotation : Scope
  L2-L3 LB Simscape : Record  FileSettingsInternal="{\"entries\":[{\"content\":{\"excelSettings\":{\"content\":{},\"type\":\"Streamout.ExcelSettings\"}},\"type\":\"Streamout.FileSettingStorage\",\"uuid\":\"ebb8c812-f4e5-4f1b-bb26-5cc9383d42b0\"}],\"packageUris\":[\"http://schema.mathworks.com/mf0/streamout_blocks/R2020a\"],\"version\":\"1.0\"}"  Layout=[1 1]  SignalsInternal="{\"entries\":[{\"content\":{\"signals\":[{\"content\":{\"blockPath\":[\"RBDmodel/L2-L3 LB readings/L2-L3 LB Simscape\"],\"dimensions\":[1],\"domain\":\"RBDmodel/L2-L3 LB readings/L2-L3 LB Simscape\",\"lineColor\":\"#fe330a\",\"port\":1,\"sid\":[\"\"],\"signalID\":1432,\"signalName\":\"L2-L3 LB Simscape Rotation\"},\"type\":\"RecordBlkView.Signal\",\"uuid\":\"e4000fb2-1268-4d0b-8a6e-88f4c6d4bada\"},{\"content\":{\"blockPath\":[\"RBDmodel/L2-L3 LB readings/L2-L3 LB Simscape\"],\"dimensions\":[1],\"domain\":\"RBDmodel/L2-L3 LB readings/L2-L3 LB Simscape\",\"lineColor\":\"#22b573\",\"port\":2,\"sid\":[\"\"],\"signalID\":1436,\"signalName\":\"L2-L3 LB Simscape Moment\"},\"type\":\"RecordBlkView.Signal\",\"uuid\":\"f21436cf-a5c5-4106-8478-03c3efb093c0\"}]},\"type\":\"RecordBlkView.InputSignals\",\"uuid\":\"bd3818c0-600a-4ad7-bacc-030b419fa0b8\"}],\"packageUris\":[\"http://schema.mathworks.com/mf0/streamout_blocks/R2020a\"],\"version\":\"1.0\"}"  VisualizationBindings="{\"xyplotplugin\":{\"info\":[{\"series\":[],\"subplotID\":1}]}}"  CompatibilityTag=XY
  wires:
  L2-L3 LB Simscape Rotation/1 -> L2-L3 LB Simscape/1, L2-L3 LB Rotation/1
  L2-L3 LB Simscape Moment/1 -> L2-L3 LB Simscape/2, L2-L3 LB Moment/1

== system RBDmodel/L3-L4 AR readings ==
  L3-L4 AR Simscape Rotation : Inport
  L3-L4 AR Simscape Moment : Inport  Port=2
  L3-L4 AR Moment : Scope
  L3-L4 AR Rotation : Scope
  L3-L4 AR Simscape : Record  FileSettingsInternal="{\"entries\":[{\"content\":{\"excelSettings\":{\"content\":{},\"type\":\"Streamout.ExcelSettings\"}},\"type\":\"Streamout.FileSettingStorage\",\"uuid\":\"0d852f55-8e65-459e-b217-a04e03d20f27\"}],\"packageUris\":[\"http://schema.mathworks.com/mf0/streamout_blocks/R2020a\"],\"version\":\"1.0\"}"  Layout=[1 1]  SignalsInternal="{\"entries\":[{\"content\":{\"signals\":[{\"content\":{\"blockPath\":[\"RBDmodel/L3-L4 AR readings/L3-L4 AR Simscape\"],\"dimensions\":[1],\"domain\":\"RBDmodel/L3-L4 AR readings/L3-L4 AR Simscape\",\"lineColor\":\"#0072bd\",\"port\":1,\"sid\":[\"\"],\"signalID\":1440,\"signalName\":\"L3-L4 AR Simscape Rotation\"},\"type\":\"RecordBlkView.Signal\",\"uuid\":\"6c4a5bfc-c544-4fcf-800c-a5faccc6cca7\"},{\"content\":{\"blockPath\":[\"RBDmodel/L3-L4 AR readings/L3-L4 AR Simscape\"],\"dimensions\":[1],\"domain\":\"RBDmodel/L3-L4 AR readings/L3-L4 AR Simscape\",\"lineColor\":\"#d95319\",\"port\":2,\"sid\":[\"\"],\"signalID\":1444,\"signalName\":\"L3-L4 AR Simscape Moment\"},\"type\":\"RecordBlkView.Signal\",\"uuid\":\"13bcb501-7d5c-4dbf-9296-921008f91faf\"}]},\"type\":\"RecordBlkView.InputSignals\",\"uuid\":\"8e96b425-26d0-473a-8dcd-ccb0931fa35b\"}],\"packageUris\":[\"http://schema.mathworks.com/mf0/streamout_blocks/R2020a\"],\"version\":\"1.0\"}"  VisualizationBindings="{\"xyplotplugin\":{\"info\":[{\"series\":[],\"subplotID\":1}]}}"  CompatibilityTag=XY
  wires:
  L3-L4 AR Simscape Rotation/1 -> L3-L4 AR Simscape/1, L3-L4 AR Rotation/1
  L3-L4 AR Simscape Moment/1 -> L3-L4 AR Simscape/2, L3-L4 AR Moment/1

== system RBDmodel/L3-L4 FE readings ==
  L3-L4 FE Simscape Rotation : Inport
  L3-L4 FE Simscape Moment : Inport  Port=2
  L3-L4 FE Moment : Scope
  L3-L4 FE Rotation : Scope
  L3-L4 FE Simscape : Record  FileSettingsInternal="{\"entries\":[{\"content\":{\"excelSettings\":{\"content\":{},\"type\":\"Streamout.ExcelSettings\"}},\"type\":\"Streamout.FileSettingStorage\",\"uuid\":\"4a97007c-b2c5-4a2b-a22c-db91ba4f89a2\"}],\"packageUris\":[\"http://schema.mathworks.com/mf0/streamout_blocks/R2020a\"],\"version\":\"1.0\"}"  Layout=[1 1]  SignalsInternal="{\"entries\":[{\"content\":{\"signals\":[{\"content\":{\"blockPath\":[\"RBDmodel/L3-L4 FE readings/L3-L4 FE Simscape\"],\"dimensions\":[1],\"domain\":\"RBDmodel/L3-L4 FE readings/L3-L4 FE Simscape\",\"lineColor\":\"#edb120\",\"port\":1,\"sid\":[\"\"],\"signalID\":1448,\"signalName\":\"L3-L4 FE Simscape Rotation\"},\"type\":\"RecordBlkView.Signal\",\"uuid\":\"db2a6a2e-7650-4c21-9b75-4aa18793a646\"},{\"content\":{\"blockPath\":[\"RBDmodel/L3-L4 FE readings/L3-L4 FE Simscape\"],\"dimensions\":[1],\"domain\":\"RBDmodel/L3-L4 FE readings/L3-L4 FE Simscape\",\"lineColor\":\"#7e2f8e\",\"port\":2,\"sid\":[\"\"],\"signalID\":1452,\"signalName\":\"L3-L4 FE Simscape Moment\"},\"type\":\"RecordBlkView.Signal\",\"uuid\":\"3957f23e-a35b-4f9b-bc33-d4b98cfad464\"}]},\"type\":\"RecordBlkView.InputSignals\",\"uuid\":\"71fa59d8-1b27-42a7-a507-b42fd9506cbb\"}],\"packageUris\":[\"http://schema.mathworks.com/mf0/streamout_blocks/R2020a\"],\"version\":\"1.0\"}"  VisualizationBindings="{\"xyplotplugin\":{\"info\":[{\"series\":[],\"subplotID\":1}]}}"  CompatibilityTag=XY
  wires:
  L3-L4 FE Simscape Rotation/1 -> L3-L4 FE Simscape/1, L3-L4 FE Rotation/1
  L3-L4 FE Simscape Moment/1 -> L3-L4 FE Simscape/2, L3-L4 FE Moment/1

== system RBDmodel/L3-L4 LB readings ==
  L3-L4 LB Simscape Rotation : Inport
  L3-L4 LB Simscape Moment : Inport  Port=2
  L3-L4 LB Moment : Scope
  L3-L4 LB Rotation : Scope
  L3-L4 LB Simscape : Record  FileSettingsInternal="{\"entries\":[{\"content\":{\"excelSettings\":{\"content\":{},\"type\":\"Streamout.ExcelSettings\"}},\"type\":\"Streamout.FileSettingStorage\",\"uuid\":\"1c058524-eb60-4b6f-8fef-1b5d5278ec82\"}],\"packageUris\":[\"http://schema.mathworks.com/mf0/streamout_blocks/R2020a\"],\"version\":\"1.0\"}"  Layout=[1 1]  SignalsInternal="{\"entries\":[{\"content\":{\"signals\":[{\"content\":{\"blockPath\":[\"RBDmodel/L3-L4 LB readings/L3-L4 LB Simscape\"],\"dimensions\":[1],\"domain\":\"RBDmodel/L3-L4 LB readings/L3-L4 LB Simscape\",\"lineColor\":\"#77ac30\",\"port\":1,\"sid\":[\"\"],\"signalID\":1456,\"signalName\":\"L3-L4 LB Simscape Rotation\"},\"type\":\"RecordBlkView.Signal\",\"uuid\":\"b8db095f-240a-43d0-84e7-d38252b604f9\"},{\"content\":{\"blockPath\":[\"RBDmodel/L3-L4 LB readings/L3-L4 LB Simscape\"],\"dimensions\":[1],\"domain\":\"RBDmodel/L3-L4 LB readings/L3-L4 LB Simscape\",\"lineColor\":\"#4dbeee\",\"port\":2,\"sid\":[\"\"],\"signalID\":1460,\"signalName\":\"L3-L4 LB Simscape Moment\"},\"type\":\"RecordBlkView.Signal\",\"uuid\":\"5b202dbb-000c-4a9c-b008-1d5c0200230d\"}]},\"type\":\"RecordBlkView.InputSignals\",\"uuid\":\"c0c580cc-b73c-4bea-ba8a-ca01a52884c2\"}],\"packageUris\":[\"http://schema.mathworks.com/mf0/streamout_blocks/R2020a\"],\"version\":\"1.0\"}"  VisualizationBindings="{\"xyplotplugin\":{\"info\":[{\"series\":[],\"subplotID\":1}]}}"  CompatibilityTag=XY
  wires:
  L3-L4 LB Simscape Rotation/1 -> L3-L4 LB Simscape/1, L3-L4 LB Rotation/1
  L3-L4 LB Simscape Moment/1 -> L3-L4 LB Simscape/2, L3-L4 LB Moment/1

== system RBDmodel/L4-L5 AR readings ==
  L4-L5 AR Simscape Rotation : Inport
  L4-L5 AR Simscape Moment : Inport  Port=2
  L4-L5 AR Moment : Scope
  L4-L5 AR Rotation : Scope
  L4-L5 AR Simscape : Record  FileSettingsInternal="{\"entries\":[{\"content\":{\"excelSettings\":{\"content\":{},\"type\":\"Streamout.ExcelSettings\"}},\"type\":\"Streamout.FileSettingStorage\",\"uuid\":\"22ee5429-b0dc-4563-83b8-15fc97b18f1f\"}],\"packageUris\":[\"http://schema.mathworks.com/mf0/streamout_blocks/R2020a\"],\"version\":\"1.0\"}"  Layout=[1 1]  SignalsInternal="{\"entries\":[{\"content\":{\"signals\":[{\"content\":{\"blockPath\":[\"RBDmodel/L4-L5 AR readings/L4-L5 AR Simscape\"],\"dimensions\":[1],\"domain\":\"RBDmodel/L4-L5 AR readings/L4-L5 AR Simscape\",\"lineColor\":\"#a2142f\",\"port\":1,\"sid\":[\"\"],\"signalID\":1464,\"signalName\":\"L4-L5 AR Simscape Rotation\"},\"type\":\"RecordBlkView.Signal\",\"uuid\":\"422b7d89-7b75-41fa-84b6-5f38bf294244\"},{\"content\":{\"blockPath\":[\"RBDmodel/L4-L5 AR readings/L4-L5 AR Simscape\"],\"dimensions\":[1],\"domain\":\"RBDmodel/L4-L5 AR readings/L4-L5 AR Simscape\",\"lineColor\":\"#139fff\",\"port\":2,\"sid\":[\"\"],\"signalID\":1468,\"signalName\":\"L4-L5 AR Simscape Moment\"},\"type\":\"RecordBlkView.Signal\",\"uuid\":\"0189dea9-829e-4520-a21c-8cf264b0c7f7\"}]},\"type\":\"RecordBlkView.InputSignals\",\"uuid\":\"1d97755c-cbbb-4ae9-9a37-30db0fc5aa7c\"}],\"packageUris\":[\"http://schema.mathworks.com/mf0/streamout_blocks/R2020a\"],\"version\":\"1.0\"}"  VisualizationBindings="{\"xyplotplugin\":{\"info\":[{\"series\":[],\"subplotID\":1}]}}"  CompatibilityTag=XY
  wires:
  L4-L5 AR Simscape Moment/1 -> L4-L5 AR Simscape/2, L4-L5 AR Moment/1
  L4-L5 AR Simscape Rotation/1 -> L4-L5 AR Simscape/1, L4-L5 AR Rotation/1

== system RBDmodel/L4-L5 FE readings ==
  L4-L5 FE Simscape Rotation : Inport
  L4-L5 FE Simscape Moment : Inport  Port=2
  L4-L5 FE Moment : Scope
  L4-L5 FE Rotation : Scope
  L4-L5 FE Simscape : Record  FileSettingsInternal="{\"entries\":[{\"content\":{\"excelSettings\":{\"content\":{},\"type\":\"Streamout.ExcelSettings\"}},\"type\":\"Streamout.FileSettingStorage\",\"uuid\":\"f454a2f2-99ca-4f18-a30c-f3205bc0580a\"}],\"packageUris\":[\"http://schema.mathworks.com/mf0/streamout_blocks/R2020a\"],\"version\":\"1.0\"}"  Layout=[1 1]  SignalsInternal="{\"entries\":[{\"content\":{\"signals\":[{\"content\":{\"blockPath\":[\"RBDmodel/L4-L5 FE readings/L4-L5 FE Simscape\"],\"dimensions\":[1],\"domain\":\"RBDmodel/L4-L5 FE readings/L4-L5 FE Simscape\",\"lineColor\":\"#ff6929\",\"port\":1,\"sid\":[\"\"],\"signalID\":1472,\"signalName\":\"L4-L5 FE Simscape Rotation\"},\"type\":\"RecordBlkView.Signal\",\"uuid\":\"14c9fac3-1bca-4e41-b574-19328547a432\"},{\"content\":{\"blockPath\":[\"RBDmodel/L4-L5 FE readings/L4-L5 FE Simscape\"],\"dimensions\":[1],\"domain\":\"RBDmodel/L4-L5 FE readings/L4-L5 FE Simscape\",\"lineColor\":\"#b746ff\",\"port\":2,\"sid\":[\"\"],\"signalID\":1476,\"signalName\":\"L4-L5 FE Simscape Moment\"},\"type\":\"RecordBlkView.Signal\",\"uuid\":\"1df36c12-5389-4755-a2f0-2cbc921b065b\"}]},\"type\":\"RecordBlkView.InputSignals\",\"uuid\":\"e4bc3aa3-f8e6-47a6-b68e-e4e3c4ed16d0\"}],\"packageUris\":[\"http://schema.mathworks.com/mf0/streamout_blocks/R2020a\"],\"version\":\"1.0\"}"  VisualizationBindings="{\"xyplotplugin\":{\"info\":[{\"series\":[],\"subplotID\":1}]}}"  CompatibilityTag=XY
  wires:
  L4-L5 FE Simscape Rotation/1 -> L4-L5 FE Simscape/1, L4-L5 FE Rotation/1
  L4-L5 FE Simscape Moment/1 -> L4-L5 FE Simscape/2, L4-L5 FE Moment/1

== system RBDmodel/L4-L5 LB readings ==
  L4-L5 LB Simscape Rotation : Inport
  L4-L5 LB Simscape Moment : Inport  Port=2
  L4-L5 LB Moment : Scope
  L4-L5 LB Rotation : Scope
  L4-L5 LB Simscape : Record  FileSettingsInternal="{\"entries\":[{\"content\":{\"excelSettings\":{\"content\":{},\"type\":\"Streamout.ExcelSettings\"}},\"type\":\"Streamout.FileSettingStorage\",\"uuid\":\"bb960ea0-e781-41a9-8e2d-b5d562a32fcc\"}],\"packageUris\":[\"http://schema.mathworks.com/mf0/streamout_blocks/R2020a\"],\"version\":\"1.0\"}"  Layout=[1 1]  SignalsInternal="{\"entries\":[{\"content\":{\"signals\":[{\"content\":{\"blockPath\":[\"RBDmodel/L4-L5 LB readings/L4-L5 LB Simscape\"],\"dimensions\":[1],\"domain\":\"RBDmodel/L4-L5 LB readings/L4-L5 LB Simscape\",\"lineColor\":\"#64d413\",\"port\":1,\"sid\":[\"\"],\"signalID\":1480,\"signalName\":\"L4-L5 LB Simscape Rotation\"},\"type\":\"RecordBlkView.Signal\",\"uuid\":\"4a64d95d-79c0-4831-b2eb-0ff7cb8b05c1\"},{\"content\":{\"blockPath\":[\"RBDmodel/L4-L5 LB readings/L4-L5 LB Simscape\"],\"dimensions\":[1],\"domain\":\"RBDmodel/L4-L5 LB readings/L4-L5 LB Simscape\",\"lineColor\":\"#ff13a6\",\"port\":2,\"sid\":[\"\"],\"signalID\":1484,\"signalName\":\"L4-L5 LB Simscape Moment\"},\"type\":\"RecordBlkView.Signal\",\"uuid\":\"c1d533e6-6e49-4d7a-9be3-a09e18e2f187\"}]},\"type\":\"RecordBlkView.InputSignals\",\"uuid\":\"7cf7667c-086e-4bc4-8afd-90e065b5399a\"}],\"packageUris\":[\"http://schema.mathworks.com/mf0/streamout_blocks/R2020a\"],\"version\":\"1.0\"}"  VisualizationBindings="{\"xyplotplugin\":{\"info\":[{\"series\":[],\"subplotID\":1}]}}"  CompatibilityTag=XY
  wires:
  L4-L5 LB Simscape Moment/1 -> L4-L5 LB Simscape/2, L4-L5 LB Moment/1
  L4-L5 LB Simscape Rotation/1 -> L4-L5 LB Simscape/1, L4-L5 LB Rotation/1

== system RBDmodel/L5-S1 AR readings ==
  L5-S1 AR Simscape Rotation : Inport
  L5-S1 AR Simscape Moment : Inport  Port=2
  L5-S1 AR Moment : Scope
  L5-S1 AR Rotation : Scope
  L5-S1 AR Simscape : Record  FileSettingsInternal="{\"entries\":[{\"content\":{\"excelSettings\":{\"content\":{},\"type\":\"Streamout.ExcelSettings\"}},\"type\":\"Streamout.FileSettingStorage\",\"uuid\":\"0ea696ca-752a-4f49-aa19-aaf05f026397\"}],\"packageUris\":[\"http://schema.mathworks.com/mf0/streamout_blocks/R2020a\"],\"version\":\"1.0\"}"  Layout=[1 1]  SignalsInternal="{\"entries\":[{\"content\":{\"signals\":[{\"content\":{\"blockPath\":[\"RBDmodel/L5-S1 AR readings/L5-S1 AR Simscape\"],\"dimensions\":[1],\"domain\":\"RBDmodel/L5-S1 AR readings/L5-S1 AR Simscape\",\"lineColor\":\"#fe330a\",\"port\":1,\"sid\":[\"\"],\"signalID\":1488,\"signalName\":\"L5-S1 AR Simscape Rotation\"},\"type\":\"RecordBlkView.Signal\",\"uuid\":\"c27297d7-5799-4c27-b00c-453bfaaa1b19\"},{\"content\":{\"blockPath\":[\"RBDmodel/L5-S1 AR readings/L5-S1 AR Simscape\"],\"dimensions\":[1],\"domain\":\"RBDmodel/L5-S1 AR readings/L5-S1 AR Simscape\",\"lineColor\":\"#22b573\",\"port\":2,\"sid\":[\"\"],\"signalID\":1492,\"signalName\":\"L5-S1 AR Simscape Moment\"},\"type\":\"RecordBlkView.Signal\",\"uuid\":\"07869cdb-c39d-4b56-9703-ab9e6bc6fe50\"}]},\"type\":\"RecordBlkView.InputSignals\",\"uuid\":\"bea89543-3d36-4a85-b080-64646e495213\"}],\"packageUris\":[\"http://schema.mathworks.com/mf0/streamout_blocks/R2020a\"],\"version\":\"1.0\"}"  VisualizationBindings="{\"xyplotplugin\":{\"info\":[{\"series\":[],\"subplotID\":1}]}}"  CompatibilityTag=XY
  wires:
  L5-S1 AR Simscape Rotation/1 -> L5-S1 AR Simscape/1, L5-S1 AR Rotation/1
  L5-S1 AR Simscape Moment/1 -> L5-S1 AR Simscape/2, L5-S1 AR Moment/1

== system RBDmodel/L5-S1 FE readings ==
  L5-S1 FE Simscape Rotation : Inport
  L5-S1 FE Simscape Moment : Inport  Port=2
  L5-S1 FE M-R : Record  FileSettingsInternal="{\"entries\":[{\"content\":{\"excelSettings\":{\"content\":{},\"type\":\"Streamout.ExcelSettings\"}},\"type\":\"Streamout.FileSettingStorage\",\"uuid\":\"03ebff2b-1b06-4da9-8d86-58934dddd7ed\"}],\"packageUris\":[\"http://schema.mathworks.com/mf0/streamout_blocks/R2020a\"],\"version\":\"1.0\"}"  Layout=[1 1]  SignalsInternal="{\"entries\":[{\"content\":{\"signals\":[{\"content\":{\"blockPath\":[\"RBDmodel/L5-S1 FE readings/L5-S1 FE M-R\"],\"dimensions\":[1],\"domain\":\"RBDmodel/L5-S1 FE readings/L5-S1 FE M-R\",\"lineColor\":\"#0072bd\",\"port\":1,\"sid\":[\"\"],\"signalID\":1496,\"signalName\":\"L5-S1 FE Simscape Rotation\"},\"type\":\"RecordBlkView.Signal\",\"uuid\":\"2ec6c761-42e8-49c8-9c9a-b5fe7ceea6b8\"},{\"content\":{\"blockPath\":[\"RBDmodel/L5-S1 FE readings/L5-S1 FE M-R\"],\"dimensions\":[1],\"domain\":\"RBDmodel/L5-S1 FE readings/L5-S1 FE M-R\",\"lineColor\":\"#d95319\",\"port\":2,\"sid\":[\"\"],\"signalID\":1500,\"signalName\":\"L5-S1 FE Simscape Moment\"},\"type\":\"RecordBlkView.Signal\",\"uuid\":\"c8e0d241-f37b-487b-b354-ea71164a3b83\"}]},\"type\":\"RecordBlkView.InputSignals\",\"uuid\":\"13376314-4a5b-4f87-961f-635f1f9372ae\"}],\"packageUris\":[\"http://schema.mathworks.com/mf0/streamout_blocks/R2020a\"],\"version\":\"1.0\"}"  VisualizationBindings="{\"xyplotplugin\":{\"info\":[{\"series\":[],\"subplotID\":1}]}}"  CompatibilityTag=XY
  L5-S1 FE Moment : Scope
  L5-S1 FE Rot : Scope
  wires:
  L5-S1 FE Simscape Rotation/1 -> L5-S1 FE M-R/1, L5-S1 FE Rot/1
  L5-S1 FE Simscape Moment/1 -> L5-S1 FE M-R/2, L5-S1 FE Moment/1

== system RBDmodel/L5-S1 LB readings ==
  L5-S1 LB Simscape Rotation : Inport
  L5-S1 LB Simscape Moment : Inport  Port=2
  L5-S1 LB Moment : Scope
  L5-S1 LB Rotation : Scope
  L5-S1 LB Simscape : Record  FileSettingsInternal="{\"entries\":[{\"content\":{\"excelSettings\":{\"content\":{},\"type\":\"Streamout.ExcelSettings\"}},\"type\":\"Streamout.FileSettingStorage\",\"uuid\":\"1fe1a201-205f-45ed-a2ea-47484a7c7520\"}],\"packageUris\":[\"http://schema.mathworks.com/mf0/streamout_blocks/R2020a\"],\"version\":\"1.0\"}"  Layout=[1 1]  SignalsInternal="{\"entries\":[{\"content\":{\"signals\":[{\"content\":{\"blockPath\":[\"RBDmodel/L5-S1 LB readings/L5-S1 LB Simscape\"],\"dimensions\":[1],\"domain\":\"RBDmodel/L5-S1 LB readings/L5-S1 LB Simscape\",\"lineColor\":\"#edb120\",\"port\":1,\"sid\":[\"\"],\"signalID\":1504,\"signalName\":\"L5-S1 LB Simscape Rotation\"},\"type\":\"RecordBlkView.Signal\",\"uuid\":\"a295ed9e-1ab4-4f18-8b40-c65e63e201f5\"},{\"content\":{\"blockPath\":[\"RBDmodel/L5-S1 LB readings/L5-S1 LB Simscape\"],\"dimensions\":[1],\"domain\":\"RBDmodel/L5-S1 LB readings/L5-S1 LB Simscape\",\"lineColor\":\"#7e2f8e\",\"port\":2,\"sid\":[\"\"],\"signalID\":1508,\"signalName\":\"L5-S1 LB Simscape Moment\"},\"type\":\"RecordBlkView.Signal\",\"uuid\":\"2e1ad242-8f6a-4bfe-9d55-da7bf28645bf\"}]},\"type\":\"RecordBlkView.InputSignals\",\"uuid\":\"992303f1-c004-4760-8ad0-1ca7bc5a1eb1\"}],\"packageUris\":[\"http://schema.mathworks.com/mf0/streamout_blocks/R2020a\"],\"version\":\"1.0\"}"  VisualizationBindings="{\"xyplotplugin\":{\"info\":[{\"series\":[],\"subplotID\":1}]}}"  CompatibilityTag=XY
  wires:
  L5-S1 LB Simscape Moment/1 -> L5-S1 LB Simscape/2, L5-S1 LB Moment/1
  L5-S1 LB Simscape Rotation/1 -> L5-S1 LB Simscape/1, L5-S1 LB Rotation/1

== system RBDmodel/Left ITL Readings ==
  In1 : Inport
  In2 : Inport  Port=2
  In3 : Inport  Port=3
  In4 : Inport  Port=4
  In5 : Inport  Port=5
  Left L1-L2 ITL force : Scope
  Left L2-L3 ITL force : Scope
  Left L4-L5 ITL force : Scope
  Left L5-S1 ITL force : Scope
  Let L3-L4 ITL force : Scope
  wires:
  In4/1 -> Left L4-L5 ITL force/1
  In1/1 -> Left L1-L2 ITL force/1
  In5/1 -> Let L3-L4 ITL force/1
  In3/1 -> Left L5-S1 ITL force/1
  In2/1 -> Left L2-L3 ITL force/1

== system RBDmodel/Muscle force inputs ==
  Area in mm^2 : Constant  Value=26819
  Constant : Constant  Value=100000
  Display : Display
  Divide : Product  Inputs=**/
  IAP in Pascals : Constant  Value=IAP_Pa
  Left Abdominal Muscle Force : Constant  Value=-LeftAbdominalMuscleForce
  Left Back Muscle Force : Constant  Value=-LeftBackMuscleForce
  Left Transverse1 Muscle Force : Constant  Value=-LeftTransverse1MuscleForce
  Left Transverse2 Muscle Force : Constant  Value=-LeftTransverse2MuscleForce
  Right Abdominal Muscle Force : Constant  Value=-RightAbdominalMuscleForce
  Right Back Muscle Force : Constant  Value=-RightBackMuscleForce
  Right Transverse1 Muscle Force : Constant  Value=-RightTransverse1MuscleForce
  Right Transverse2 Muscle Force : Constant  Value=-RightTransverse2MuscleForce
  Scope{1..8} (8 alike) : Scope
  Sum of Square of Forces : MATLAB Function  TreatAsAtomicUnit=on
  RightAbdominalMuscleForce : Outport
  LeftAbdominalMuscleForce : Outport  Port=2
  RightBackMuscleForce : Outport  Port=3
  LeftBackMuscleForce : Outport  Port=4
  RightTransverse1MuscleForce : Outport  Port=5
  RightTransverse2MuscleForce : Outport  Port=6
  LeftTransverse1MuscleForce : Outport  Port=7
  LeftTransverse2MuscleForce : Outport  Port=8
  wires:
  Left Transverse2 Muscle Force/1 -> LeftTransverse2MuscleForce/1, Scope8/1, Sum of Square of Forces/8(F8)  "LeftTransverse2MuscleForce"
  Left Abdominal Muscle Force/1 -> LeftAbdominalMuscleForce/1, Scope2/1, Sum of Square of Forces/2(F2)  "LeftAbdominalMuscleForce"
  Sum of Square of Forces/1(SumofSquareofForces) -> Display/1  "SumofSquareofForces"
  Area in mm^2/1 -> Divide/2
  Left Back Muscle Force/1 -> Sum of Square of Forces/4(F4), LeftBackMuscleForce/1, Scope4/1  "LeftBackMuscleForce"
  Divide/1 -> Sum of Square of Forces/9(IAP)
  Left Transverse1 Muscle Force/1 -> LeftTransverse1MuscleForce/1, Scope7/1, Sum of Square of Forces/6(F6)  "LeftTransverse1MuscleForce"
  Right Abdominal Muscle Force/1 -> RightAbdominalMuscleForce/1, Scope1/1, Sum of Square of Forces/1(F1)  "RightAbdominalMuscleForce"
  Right Back Muscle Force/1 -> RightBackMuscleForce/1, Scope3/1, Sum of Square of Forces/3(F3)  "RightBackMuscleForce"
  Right Transverse2 Muscle Force/1 -> RightTransverse2MuscleForce/1, Scope6/1, Sum of Square of Forces/5(F5)  "RightTransverse2MuscleForce"
  Right Transverse1 Muscle Force/1 -> RightTransverse1MuscleForce/1, Scope5/1, Sum of Square of Forces/7(F7)  "RightTransverse1MuscleForce"
  IAP in Pascals/1 -> Divide/1
  Constant/1 -> Divide/3

== system RBDmodel/Plumbline readings ==
  x : Inport
  y : Inport  Port=2
  z : Inport  Port=3
  Check X Bounds : checkpacklib/Check Custom Bounds  InstantiateOnLoad=on  enabled=off  stopWhenAssertionFail=off  export=off  ViewDlgPos=[983.4 172.2 510.4 379.2]  OpenViewOnLoad=off  LaunchViewOnOpen=off  TimeUnits=seconds  EnableUpperBound=on  UpperBoundTimes=[0 3]  UpperBoundAmplitudes=[2 2];  EnableLowerBound=on  LowerBoundTimes=[0 3]  LowerBoundAmplitudes=[-2 -2]
      settings: LibrarySourceBlock=sdolib/Signal Constraints/Check Custom Bounds
  Check Y Bounds : checkpacklib/Check Custom Bounds  InstantiateOnLoad=on  enabled=off  stopWhenAssertionFail=off  export=off  ViewDlgPos=[509 222 510 390]  OpenViewOnLoad=off  LaunchViewOnOpen=off  TimeUnits=seconds  EnableUpperBound=on  UpperBoundTimes=[0 3]  UpperBoundAmplitudes=[2 2];  EnableLowerBound=on  LowerBoundTimes=[0 3]  LowerBoundAmplitudes=[-2 -2]
      settings: LibrarySourceBlock=sdolib/Signal Constraints/Check Custom Bounds
  Plumbline X distance (cm) : Display
  Plumbline Y distance (cm) : Display
  Plumbline Z distance (cm) : Display
  T1 plumbline coordinates : Scope  NumInputPorts=3
  wires:
  x/1 -> Plumbline X distance (cm)/1, Check X Bounds/1, T1 plumbline coordinates/1
  z/1 -> Plumbline Z distance (cm)/1, T1 plumbline coordinates/3
  y/1 -> Plumbline Y distance (cm)/1, Check Y Bounds/1, T1 plumbline coordinates/2
